simulink model "Islanding_case"  (R2024b)
settings: Solver=ode3  StartTime=0.0  StopTime=2.8  FixedStep=Ts  RelTol=1e-3  EnableMultiTasking=on
InitFcn:
  | Ts=100e-6;
  | Ts_Control=100e-6;
  | Ts_Power=100e-6;
  | tvv=0.1;
  | tr=1;
  | RelayEnableTime=1;
  | En_MC=1;
  | 
  | % ================= CHOOSE THE CASE HERE ==================
  | CaseNo    = 1;      % 1 = grid connected   2 = islanding   3 = fault during islanding
  | FaultType = 'none';   % 'none'  'LG'  'LL'  'LLG'  'LLL'  'LLLG'   (not used in case 2)
  | Qmismatch = 0;      % extra capacitive reactive power (% of 1.5 MW per load); try 1 in case 2 to see the inverter trip
  | % =========================================================
  | 
  | % ---- settings derived from the case (no need to edit)
  | switch CaseNo
  |     case 1, Tisland = 100; Pmismatch = 50; Tf = 2.0;   % grid + PV supply the load, fault at 2.0 s
  |     case 2, Tisland = 2.0; Pmismatch = 0;  Tf = 100;   % breakers open at 2.0 s, no fault
  |     case 3, Tisland = 2.0; Pmismatch = 0;  Tf = 2.3;   % breakers open at 2.0 s, fault at 2.3 s
  |     otherwise, error('CaseNo must be 1, 2 or 3');
  | end
  | FaultDur = 0.1;     % fault duration (s)
  | Tf_LG   = 100; Tf_LL = 100; Tf_LLG = 100; Tf_LLL = 100; Tf_LLLG = 100;   % 100 = never
  | switch upper(FaultType)
  |     case 'LG',   Tf_LG   = Tf;
  |     case 'LL',   Tf_LL   = Tf;
  |     case 'LLG',  Tf_LLG  = Tf;
  |     case 'LLL',  Tf_LLL  = Tf;
  |     case 'LLLG', Tf_LLLG = Tf;
  |     case 'NONE'
  |     otherwise, error('FaultType must be none, LG, LL, LLG, LLL or LLLG');
  | end
undefined symbols (not defined in the file or in its folder): DiscIntNeverNeededParam, Finit, Newton, Raphson, Tisland
libraries: simulink x33, spsOnDelayLib x17, powerlib_extras x11, eeGeneralControl x9, spsThreePhaseFaultLib x6, slpidlib x6, spsThreePhaseVIMeasurementLib x4, spsSampleandHoldLib x4, spsAlphaBetaZerotodq0Lib x4, spsThreePhaseSourceLib x4, spsThreePhaseBreakerLib x3, simulink_extras x3
(part 3 of 4)

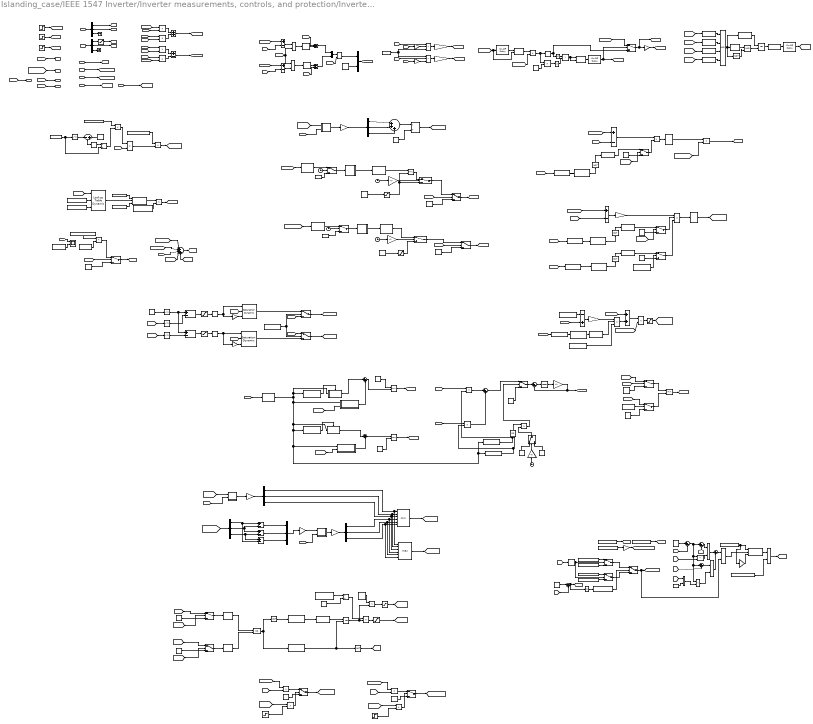
== system Islanding_case/IEEE 1547 Inverter/Inverter measurements, controls, and protection/Inverter control in positive sequence/Controls and grid support functions block ==
  note: |
      | |
      | |
      | |
      | |
      | |
      | |
      | |
      | |
      | |
      | |
      | |
      | |
      | |
      | |
      | |
      | |
      | |
      | |
      | |
      | |
      | |
      | |
      | |
      | |
      | |
      | |
      | |
      | |
      | |
      | |
      | |
      | |
      | |
      | |
      | |
      | |
      | |
      | |
      | |
      | |
      | |
      | |
      | |
      | |
      | |
      | |
      | |
      | |
      | |
      | |
      | |
      | |
      | |
      | |
      | |
  note: Group 2C Islanding Detection Function
  note: Enter Service Criteria
  note: Enter service
  note: Dynamic Voltage Support (DVS) in positive sequence
  note: Watt-Var Function
  note: Constant Q Function
  note: Constant PF Function
  note: |
      | |
      | |
      | |
      | |
      | |
      | |
      | |
      | |
      | |
      | |
      | |
      | |
      | |
      | |
      | |
      | |
      | |
      | |
      | |
  note: |
      | |
      | |
      | |
      | |
      | |
      | |
      | |
      | |
      | |
      | |
      | |
      | |
      | |
      | |
      | |
      | |
      | |
      | |
      | |
      | |
      | |
      | |
      | |
      | |
      | |
      | |
      | |
      | |
      | |
      | |
      | |
      | |
      | |
      | |
      | |
      | |
      | |
      | |
      | |
      | |
      | |
      | |
      | |
      | |
      | |
      | |
      | |
      | |
      | |
      | |
      | |
      | |
      | |
      | |
      | |
  note: Vca_rms
  note: Vbc_rms
  note: Vab_rms
  note: Vb_rms
  note: Vc_rms
  note: Vab
  note: Vca
  note: Vbc
  note: Va_rms
  note: If Volt-Var function is turned off, the inverter will function at unity power factor
  note: Momentary Cessation recover signal reset. Reset is 0 when momentary cessation ends and 1 during momentary cessation
  note: Volt-Var curve points
  note: Volt-watt curve points
  note: Output of the freq-watt control. Control to ensure that the output is either the active power adjustment due to under or over frequency
  note: Minimum of the active power generated from freq-watt control and volt-watt control
      | (PFV is the input to the power limiter)
  note: Active power adjustment for over frequency condition
  note: Active power adjustment for under frequency condition
  note: Maximum of phase to ground and phase to phase voltages as input to Momentary Cessation
  note: Minimum of phase to ground and phase to phase voltages as input to Momentary Cessation
  note: Momentary Cessation recovery ramp rate signal for active current
  note: Combine enter and exit Momentary Cessation signal into one control signal for active current
  note: Combine enter and exit Momentary Cessation signal into one control signal for reactive current
  note: Exit Momentary Cessation signal (Must be between 0 and 1)
  note: Enter Momentary Cessation signal
      | MC_sig is 0 when enter momentary cessation otherwise MC_sig is 1
  note: Multiply current references with MC_power_control to enter and exit Momentary Cessation
  note: Input to Momentary Cessation
  note: Momentary Cessation
  note: Freq-Watt Function
  note: Input to Volt-Watt and Volt-Var Function
  note: Volt-Watt Function
  note: Volt-Var Function
  note: Power limiter with Q priority
  note: Reactive power control
  note: Active power control
  note: Current controller
  note: Power calculation
  note: |
      | |
      | |
      | |
      | |
      | |
      | |
      | |
      | |
      | |
      | |
      | |
      | |
      | |
      | |
      | |
      | |
      | |
      | |
      | |
  note: |
      | |
      | |
      | |
      | |
      | |
      | |
      | |
      | |
      | |
      | |
      | |
      | |
      | |
      | |
      | |
      | |
      | |
      | |
      | |
      | |
      | |
      | |
      | |
      | |
      | |
      | |
      | |
      | |
      | |
      | |
      | |
      | |
      | |
      | |
      | |
      | |
      | |
      | |
      | |
      | |
      | |
      | |
      | |
      | |
      | |
      | |
      | |
      | |
      | |
      | |
      | |
      | |
      | |
      | |
      | |
  note: ==============================================================================================================================================================================================================================
  note: ========================================================================================================================================================================================================================================================
  note: ========================================================================================================================================================================================================================================================
  note: |
      | |
      | |
      | |
      | |
      | |
      | |
      | |
      | |
      | |
      | |
      | |
      | |
      | |
      | |
      | |
      | |
      | |
      | |
      | |
  note: |
      | |
      | |
      | |
      | |
      | |
      | |
      | |
      | |
      | |
      | |
      | |
      | |
      | |
      | |
      | |
      | |
      | |
      | |
      | |
  note: Inputs
  note: =============================================================================================================================================================================================================================================================================
  note: Pmin
  note: Pavailable
  note: |
      | |
      | |
      | |
      | |
      | |
      | |
      | |
      | |
      | |
      | |
      | |
      | |
      | |
      | |
      | |
      | |
      | |
      | |
      | |
  I_dq : Inport
  f : Inport  Port=2
  V_dq : Inport  Port=3
  Vpccpu : Inport  Port=4
  Vpcc : Inport  Port=5
  Idref_lim : Inport  Port=6
  Iqref_lim : Inport  Port=7
  -2 : Gain  Gain=Kpos  SaturateOnIntegerOverflow=on  OutDataTypeStr=Inherit: Same as input  ParamDataTypeStr=Inherit: Same as input
  -3 : Gain  Gain=-1  SaturateOnIntegerOverflow=on  OutDataTypeStr=Inherit: Same as input  ParamDataTypeStr=Inherit: Same as input
  -kd*L_ac : Gain  Gain=-kd*L_dec  SaturateOnIntegerOverflow=on  OutDataTypeStr=Inherit: Same as input  ParamDataTypeStr=Inherit: Same as input
  81U-2 Delay : spsOnDelayLib/On Delay  DelayType=On delay  delay=.016  ic=0  Ts=0
  81U-2 Delay1 : spsOnDelayLib/On Delay  DelayType=On delay  delay=.016  ic=0  Ts=0
  81U-2 Delay3 : spsOnDelayLib/On Delay  DelayType=Off delay  delay=0.016  ic=0  Ts=0
  81U-2 Delay4 : spsOnDelayLib/On Delay  DelayType=Off delay  delay=1/MC_recoveryrate  ic=0  Ts=0
  81U-2 Delay5 : spsOnDelayLib/On Delay  DelayType=Off delay  delay=0.016  ic=0  Ts=0
  81U-2 Delay6 : spsOnDelayLib/On Delay  DelayType=Off delay  delay=0.016  ic=0  Ts=0
  AND : Logic  Inputs=4  IconShape=distinctive  AllPortsSameDT=off  OutDataTypeStr=boolean
  AND1 : Logic  IconShape=distinctive  AllPortsSameDT=off  OutDataTypeStr=boolean
  Abs : Abs  SaturateOnIntegerOverflow=off
  Abs1 : Abs  SaturateOnIntegerOverflow=off
  Abs2 : Abs  SaturateOnIntegerOverflow=off
  Activate : Product  OutDataTypeStr=double  RndMeth=Zero
  Activate1 : Product  OutDataTypeStr=double  RndMeth=Zero
  Activate3 : Product  OutDataTypeStr=double  RndMeth=Zero
  CONST_Q_MOD_ENABLE : Constant  Value=CONST_Q_MODE_ENABLE
  Clock{,1..2,5..6} (5 alike) : Clock
  Compare To Constant : simulink/Logic and Bit Operations/Compare To Constant  relop=<  const=low_MC  OutDataTypeStr=boolean
  Compare To Constant1 : simulink/Logic and Bit Operations/Compare To Constant  relop=>  const=high_MC  OutDataTypeStr=boolean
  Compare To Constant2 : simulink/Logic and Bit Operations/Compare To Constant  relop=>  const=ES_V_LOW  OutDataTypeStr=boolean
  Compare To Constant3 : simulink/Logic and Bit Operations/Compare To Constant  relop=<  const=ES_V_HIGH  OutDataTypeStr=boolean
  Compare To Constant4 : simulink/Logic and Bit Operations/Compare To Constant  relop=>  const=ES_F_LOW  OutDataTypeStr=boolean
  Compare To Constant5 : simulink/Logic and Bit Operations/Compare To Constant  relop=<  const=ES_F_HIGH  OutDataTypeStr=boolean
  Compare To Constant6 : simulink/Logic and Bit Operations/Compare To Constant  relop=>  const=ES_DELAY  OutDataTypeStr=boolean
  Compare To Constant7 : simulink/Logic and Bit Operations/Compare To Constant  relop=<=  const=NomFreq  OutDataTypeStr=boolean
  Compare To Constant8 : simulink/Logic and Bit Operations/Compare To Constant  relop=<  const=GROUP2C_AI_F_TH  OutDataTypeStr=boolean
  Const : Constant
  Constant : Constant  Value=Pmin  SampleTime=-1
  Constant{1,3,6..7,9,13,15..16,32..34} (11 alike) : Constant  SampleTime=-1
  Constant10 : Constant  Value=MC_recoveryrate  SampleTime=-1
  Constant11 : Constant  Value=1/0.016  SampleTime=-1
  Constant12 : Constant  Value=0.999
  Constant14 : Constant  Value=0  SampleTime=-1
  Constant17 : Constant  Value=-1
  Constant18 : Constant  Value=GROUP2C_AI_LIMIT
  Constant19 : Constant  Value=GROUP2C_AI_DB
  Constant2 : Constant  Value=EnableVW  SampleTime=-1
  Constant20 : Constant  Value=GROUP2C_AI_DB
  Constant21 : Constant  Value=GROUP2C_AI_LIMIT
  Constant22 : Constant  Value=GROUP2C_AI_LG1
  Constant23 : Constant  Value=GROUP2C_AI_HG1
  Constant24 : Constant  Value=GROUP2C_AI_LG2
  Constant25 : Constant  Value=GROUP2C_AI_HG2
  Constant26 : Constant  Value=NomFreq
  Constant28 : Constant  Value=GROUP2C_AI_ENABLE
  Constant30 : Constant  Value=CONST_Q_ref
  Constant31 : Constant  Value=CONST_Q_ref
  Constant4 : Constant  Value=Pref  SampleTime=-1
  Constant5 : Constant  Value=3  SampleTime=-1
  Constant8 : Constant  Value=NomFreq
  ConstantPF : Constant  Value=Constant_PF
  Constant_PF_Excitation : Constant  Value=Constant_PF_Excitation
  Constant_PF_Mode_Enable : Constant  Value=Constant_PF_Mode_Enable
  Convert to PU1 : Gain  Gain=1/((RMSVnom*sqrt(3))*sqrt(2))  SaturateOnIntegerOverflow=on  OutDataTypeStr=Inherit: Same as input  ParamDataTypeStr=Inherit: Same as input
  Data Type Conversion{,1..5} (6 alike) : DataTypeConversion  OutDataTypeStr=double  SaturateOnIntegerOverflow=off  RndMeth=Floor
  Demux{,1..2,7,9,11} (6 alike) : Demux  Outputs=3
  Discrete PID Controller : slpidlib/PID Controller  Controller=PI  Form=Parallel  TimeDomain=Continuous-time  UseExternalTs=off  SampleTime=-1  IntegratorMethod=Forward Euler  FilterMethod=Forward Euler  ControllerParametersSource=internal  P=Kpi  I=Kii  UseKiTs=off  D=0  UseExternalDerivativeSource=off  N=100  UseFilter=on  TunerSelectOption=Transfer Function Based (PID Tuner App)  InitialConditionSource=internal  InitialConditionForIntegrator=0.65  InitialConditionForFilter=0  DifferentiatorICPrevScaledInput=0  ExternalReset=none  TrackingMode=off  Kt=1  LimitOutput=on  SatLimitsSource=internal  UpperSaturationLimit=1  LowerSaturationLimit=-1  LinearizeAsGain=off  AntiWindupMode=none  Kb=1  LimitIntegrator=off  UpperIntegratorSaturationLimit=inf  LowerIntegratorSaturationLimit=-inf  POutMin=[]  POutMax=[]  IOutMin=[]  IOutMax=[]  DOutMin=[]  DOutMax=[]  NOutMin=[]  NOutMax=[]  SumOutMin=[]  SumOutMax=[]  SaturationOutMin=[]  SaturationOutMax=[]  PParamMin=[]  PParamMax=[]  IParamMin=[]  IParamMax=[]  DParamMin=[]  DParamMax=[]  NParamMin=[]  NParamMax=[]  KbParamMin=[]  KbParamMax=[]  KtParamMin=[]  KtParamMax=[]  KbOutMin=[]  KbOutMax=[]  KtOutMin=[]  KtOutMax=[]  IntegratorOutMin=[]  IntegratorOutMax=[]  FilterOutMin=[]  FilterOutMax=[]  SumI1OutMin=[]  SumI1OutMax=[]  SumI2OutMin=[]  SumI2OutMax=[]  SumI3OutMin=[]  SumI3OutMax=[]  SumI4OutMin=[]  SumI4OutMax=[]  SumDOutMin=[]  SumDOutMax=[]  DifferentiatorOutMin=[]  DifferentiatorOutMax=[]  FilterDiffOutCoefMin=[]  FilterDiffOutCoefMax=[]  ReciprocalOutMin=[]  ReciprocalOutMax=[]  SumDenOutMin=[]  SumDenOutMax=[]  SumNumOutMin=[]  SumNumOutMax=[]  DivideOutMin=[]  DivideOutMax=[]  UdiffTsProdOutMin=[]  UdiffTsProdOutMax=[]  NTsProdOutMin=[]  NTsProdOutMax=[]  UintegralTsProdOutMin=[]  UintegralTsProdOutMax=[]  UngainTsProdOutMin=[]  UngainTsProdOutMax=[]  ClampingZeroOutDataTypeStr=Inherit: Inherit via back propagation  ClampingZeroOutMin=[]  ClampingZeroOutMax=[]  FilterDenConstantOutDataTypeStr=Inherit: Inherit via back propagation  FilterDenConstantOutMin=[]  FilterDenConstantOutMax=[]  PCopyOutDataTypeStr=Inherit: Inherit via back propagation  PCopyOutMin=[]  PCopyOutMax=[]  NCopyOutDataTypeStr=Inherit: Inherit via back propagation  NCopyOutMin=[]  NCopyOutMax=[]  IntegratorContinuousStateAttributes=''  IntegratorStateMustResolveToSignalObject=off  IntegratorRTWStateStorageClass=Auto  FilterContinuousStateAttributes=''  FilterStateMustResolveToSignalObject=off  FilterRTWStateStorageClass=Auto  ParallelPVariant=InternalParameters  IdealPVariant=Disabled  IVariant=InternalParameters  DVariant=Disabled  IntegratorVariant=Continuous  SatVariant=Enabled  AWVariant=Passthrough  PCopyVariant=Disabled  TRVariant=Disabled  FdbkBlocksVariant=Forward  IdealPFdbkVariant=Disabled  SatFdbkVariant=Disabled  DerivativeFilterVariant=Disabled  NVariant=Disabled  NCopyVariant=Disabled_SignalSpec  FilterICVariant=Disabled  IntegratorICVariant=InternalICs  ExternalResetVariant=Disabled  TRSumVariant=Passthrough  SumFdbkVariant=Disabled  SumVariant=Sum_PI  TsampFilterVariant=InternalTs  TsampNgainVariant=Passthrough  TsampIntegralVariant=Disabled_SignalSpec  ExternalSaturationOutDataTypeStr=Inherit: Same as second input  DerivativeSourceVariant=Disabled  PreIntVariant=InternalPreInt
  Discrete PID Controller1 : slpidlib/PID Controller  Controller=PI  Form=Parallel  TimeDomain=Continuous-time  UseExternalTs=off  SampleTime=-1  IntegratorMethod=Forward Euler  FilterMethod=Forward Euler  ControllerParametersSource=internal  P=Kpi  I=Kii  UseKiTs=off  D=0  UseExternalDerivativeSource=off  N=100  UseFilter=on  TunerSelectOption=Transfer Function Based (PID Tuner App)  InitialConditionSource=internal  InitialConditionForIntegrator=0  InitialConditionForFilter=0  DifferentiatorICPrevScaledInput=0  ExternalReset=none  TrackingMode=off  Kt=1  LimitOutput=on  SatLimitsSource=internal  UpperSaturationLimit=1  LowerSaturationLimit=-1  LinearizeAsGain=off  AntiWindupMode=none  Kb=1  LimitIntegrator=off  UpperIntegratorSaturationLimit=inf  LowerIntegratorSaturationLimit=-inf  POutMin=[]  POutMax=[]  IOutMin=[]  IOutMax=[]  DOutMin=[]  DOutMax=[]  NOutMin=[]  NOutMax=[]  SumOutMin=[]  SumOutMax=[]  SaturationOutMin=[]  SaturationOutMax=[]  PParamMin=[]  PParamMax=[]  IParamMin=[]  IParamMax=[]  DParamMin=[]  DParamMax=[]  NParamMin=[]  NParamMax=[]  KbParamMin=[]  KbParamMax=[]  KtParamMin=[]  KtParamMax=[]  KbOutMin=[]  KbOutMax=[]  KtOutMin=[]  KtOutMax=[]  IntegratorOutMin=[]  IntegratorOutMax=[]  FilterOutMin=[]  FilterOutMax=[]  SumI1OutMin=[]  SumI1OutMax=[]  SumI2OutMin=[]  SumI2OutMax=[]  SumI3OutMin=[]  SumI3OutMax=[]  SumI4OutMin=[]  SumI4OutMax=[]  SumDOutMin=[]  SumDOutMax=[]  DifferentiatorOutMin=[]  DifferentiatorOutMax=[]  FilterDiffOutCoefMin=[]  FilterDiffOutCoefMax=[]  ReciprocalOutMin=[]  ReciprocalOutMax=[]  SumDenOutMin=[]  SumDenOutMax=[]  SumNumOutMin=[]  SumNumOutMax=[]  DivideOutMin=[]  DivideOutMax=[]  UdiffTsProdOutMin=[]  UdiffTsProdOutMax=[]  NTsProdOutMin=[]  NTsProdOutMax=[]  UintegralTsProdOutMin=[]  UintegralTsProdOutMax=[]  UngainTsProdOutMin=[]  UngainTsProdOutMax=[]  ClampingZeroOutDataTypeStr=Inherit: Inherit via back propagation  ClampingZeroOutMin=[]  ClampingZeroOutMax=[]  FilterDenConstantOutDataTypeStr=Inherit: Inherit via back propagation  FilterDenConstantOutMin=[]  FilterDenConstantOutMax=[]  PCopyOutDataTypeStr=Inherit: Inherit via back propagation  PCopyOutMin=[]  PCopyOutMax=[]  NCopyOutDataTypeStr=Inherit: Inherit via back propagation  NCopyOutMin=[]  NCopyOutMax=[]  IntegratorContinuousStateAttributes=''  IntegratorStateMustResolveToSignalObject=off  IntegratorRTWStateStorageClass=Auto  FilterContinuousStateAttributes=''  FilterStateMustResolveToSignalObject=off  FilterRTWStateStorageClass=Auto  ParallelPVariant=InternalParameters  IdealPVariant=Disabled  IVariant=InternalParameters  DVariant=Disabled  IntegratorVariant=Continuous  SatVariant=Enabled  AWVariant=Passthrough  PCopyVariant=Disabled  TRVariant=Disabled  FdbkBlocksVariant=Forward  IdealPFdbkVariant=Disabled  SatFdbkVariant=Disabled  DerivativeFilterVariant=Disabled  NVariant=Disabled  NCopyVariant=Disabled_SignalSpec  FilterICVariant=Disabled  IntegratorICVariant=InternalICs  ExternalResetVariant=Disabled  TRSumVariant=Passthrough  SumFdbkVariant=Disabled  SumVariant=Sum_PI  TsampFilterVariant=InternalTs  TsampNgainVariant=Passthrough  TsampIntegralVariant=Disabled_SignalSpec  ExternalSaturationOutDataTypeStr=Inherit: Same as second input  DerivativeSourceVariant=Disabled  PreIntVariant=InternalPreInt
  Discrete PID Controller3 : slpidlib/PID Controller  Controller=PI  Form=Parallel  TimeDomain=Discrete-time  UseExternalTs=off  SampleTime=-1  IntegratorMethod=Backward Euler  FilterMethod=Forward Euler  ControllerParametersSource=internal  P=Kpp  I=Kip  UseKiTs=off  D=0  UseExternalDerivativeSource=off  N=100  UseFilter=on  TunerSelectOption=Transfer Function Based (PID Tuner App)  ZeroCross=off  InitialConditionSource=internal  InitialConditionForIntegrator=0  InitialConditionForFilter=0  DifferentiatorICPrevScaledInput=0  ExternalReset=none  TrackingMode=off  Kt=1  LimitOutput=on  SatLimitsSource=internal  UpperSaturationLimit=Imax  LowerSaturationLimit=-Imax  LinearizeAsGain=off  AntiWindupMode=back-calculation  Kb=1  LimitIntegrator=off  UpperIntegratorSaturationLimit=inf  LowerIntegratorSaturationLimit=-inf  POutMin=[]  POutMax=[]  IOutMin=[]  IOutMax=[]  DOutMin=[]  DOutMax=[]  NOutMin=[]  NOutMax=[]  SumOutMin=[]  SumOutMax=[]  SaturationOutMin=[]  SaturationOutMax=[]  PParamMin=[]  PParamMax=[]  IParamMin=[]  IParamMax=[]  DParamMin=[]  DParamMax=[]  NParamMin=[]  NParamMax=[]  KbParamMin=[]  KbParamMax=[]  KtParamMin=[]  KtParamMax=[]  KbOutMin=[]  KbOutMax=[]  KtOutMin=[]  KtOutMax=[]  IntegratorOutMin=[]  IntegratorOutMax=[]  FilterOutMin=[]  FilterOutMax=[]  SumI1OutMin=[]  SumI1OutMax=[]  SumI2OutMin=[]  SumI2OutMax=[]  SumI3OutMin=[]  SumI3OutMax=[]  SumI4OutMin=[]  SumI4OutMax=[]  SumDOutMin=[]  SumDOutMax=[]  DifferentiatorOutMin=[]  DifferentiatorOutMax=[]  FilterDiffOutCoefMin=[]  FilterDiffOutCoefMax=[]  ReciprocalOutMin=[]  ReciprocalOutMax=[]  SumDenOutMin=[]  SumDenOutMax=[]  SumNumOutMin=[]  SumNumOutMax=[]  DivideOutMin=[]  DivideOutMax=[]  UdiffTsProdOutMin=[]  UdiffTsProdOutMax=[]  NTsProdOutMin=[]  NTsProdOutMax=[]  UintegralTsProdOutMin=[]  UintegralTsProdOutMax=[]  UngainTsProdOutMin=[]  UngainTsProdOutMax=[]  ClampingZeroOutDataTypeStr=Inherit: Inherit via back propagation  ClampingZeroOutMin=[]  ClampingZeroOutMax=[]  FilterDenConstantOutDataTypeStr=Inherit: Inherit via back propagation  FilterDenConstantOutMin=[]  FilterDenConstantOutMax=[]  PCopyOutDataTypeStr=Inherit: Inherit via back propagation  PCopyOutMin=[]  PCopyOutMax=[]  NCopyOutDataTypeStr=Inherit: Inherit via back propagation  NCopyOutMin=[]  NCopyOutMax=[]  IntegratorContinuousStateAttributes=''  IntegratorStateMustResolveToSignalObject=off  IntegratorRTWStateStorageClass=Auto  FilterContinuousStateAttributes=''  FilterStateMustResolveToSignalObject=off  FilterRTWStateStorageClass=Auto  ParallelPVariant=InternalParameters  IdealPVariant=Disabled  IVariant=InternalParameters  DVariant=Disabled  IntegratorVariant=Discrete  SatVariant=Enabled  AWVariant=BackCalculation  PCopyVariant=Disabled  TRVariant=Disabled  FdbkBlocksVariant=Feedback  IdealPFdbkVariant=Passthrough  SatFdbkVariant=Enabled  DerivativeFilterVariant=Disabled  NVariant=Disabled  NCopyVariant=Disabled_SignalSpec  FilterICVariant=Disabled  IntegratorICVariant=InternalICs  ExternalResetVariant=Disabled  TRSumVariant=Passthrough  SumFdbkVariant=Enabled  SumVariant=Sum_PI  TsampFilterVariant=InternalTs  TsampNgainVariant=Passthrough  TsampIntegralVariant=Disabled_SignalSpec  ExternalSaturationOutDataTypeStr=Inherit: Same as second input  DerivativeSourceVariant=Disabled  PreIntVariant=InternalPreInt
  Discrete PID Controller6 : slpidlib/PID Controller  Controller=PI  Form=Parallel  TimeDomain=Discrete-time  UseExternalTs=off  SampleTime=-1  IntegratorMethod=Backward Euler  FilterMethod=Forward Euler  ControllerParametersSource=internal  P=Kpp  I=Kip  UseKiTs=off  D=0  UseExternalDerivativeSource=off  N=100  UseFilter=on  TunerSelectOption=Transfer Function Based (PID Tuner App)  ZeroCross=off  InitialConditionSource=internal  InitialConditionForIntegrator=0  InitialConditionForFilter=0  DifferentiatorICPrevScaledInput=0  ExternalReset=none  TrackingMode=off  Kt=1  LimitOutput=on  SatLimitsSource=internal  UpperSaturationLimit=Imax  LowerSaturationLimit=-Imax  LinearizeAsGain=off  AntiWindupMode=clamping  Kb=1  LimitIntegrator=off  UpperIntegratorSaturationLimit=inf  LowerIntegratorSaturationLimit=-inf  POutMin=[]  POutMax=[]  IOutMin=[]  IOutMax=[]  DOutMin=[]  DOutMax=[]  NOutMin=[]  NOutMax=[]  SumOutMin=[]  SumOutMax=[]  SaturationOutMin=[]  SaturationOutMax=[]  PParamMin=[]  PParamMax=[]  IParamMin=[]  IParamMax=[]  DParamMin=[]  DParamMax=[]  NParamMin=[]  NParamMax=[]  KbParamMin=[]  KbParamMax=[]  KtParamMin=[]  KtParamMax=[]  KbOutMin=[]  KbOutMax=[]  KtOutMin=[]  KtOutMax=[]  IntegratorOutMin=[]  IntegratorOutMax=[]  FilterOutMin=[]  FilterOutMax=[]  SumI1OutMin=[]  SumI1OutMax=[]  SumI2OutMin=[]  SumI2OutMax=[]  SumI3OutMin=[]  SumI3OutMax=[]  SumI4OutMin=[]  SumI4OutMax=[]  SumDOutMin=[]  SumDOutMax=[]  DifferentiatorOutMin=[]  DifferentiatorOutMax=[]  FilterDiffOutCoefMin=[]  FilterDiffOutCoefMax=[]  ReciprocalOutMin=[]  ReciprocalOutMax=[]  SumDenOutMin=[]  SumDenOutMax=[]  SumNumOutMin=[]  SumNumOutMax=[]  DivideOutMin=[]  DivideOutMax=[]  UdiffTsProdOutMin=[]  UdiffTsProdOutMax=[]  NTsProdOutMin=[]  NTsProdOutMax=[]  UintegralTsProdOutMin=[]  UintegralTsProdOutMax=[]  UngainTsProdOutMin=[]  UngainTsProdOutMax=[]  ClampingZeroOutDataTypeStr=Inherit: Inherit via back propagation  ClampingZeroOutMin=[]  ClampingZeroOutMax=[]  FilterDenConstantOutDataTypeStr=Inherit: Inherit via back propagation  FilterDenConstantOutMin=[]  FilterDenConstantOutMax=[]  PCopyOutDataTypeStr=Inherit: Inherit via back propagation  PCopyOutMin=[]  PCopyOutMax=[]  NCopyOutDataTypeStr=Inherit: Inherit via back propagation  NCopyOutMin=[]  NCopyOutMax=[]  IntegratorContinuousStateAttributes=''  IntegratorStateMustResolveToSignalObject=off  IntegratorRTWStateStorageClass=Auto  FilterContinuousStateAttributes=''  FilterStateMustResolveToSignalObject=off  FilterRTWStateStorageClass=Auto  ParallelPVariant=InternalParameters  IdealPVariant=Disabled  IVariant=InternalParameters  DVariant=Disabled  IntegratorVariant=Discrete  SatVariant=Enabled  AWVariant=DiscClampingParallel  PCopyVariant=Disabled  TRVariant=Disabled  FdbkBlocksVariant=Feedback  IdealPFdbkVariant=Passthrough  SatFdbkVariant=Passthrough  DerivativeFilterVariant=Disabled  NVariant=Disabled  NCopyVariant=Disabled_SignalSpec  FilterICVariant=Disabled  IntegratorICVariant=InternalICs  ExternalResetVariant=Disabled  TRSumVariant=Passthrough  SumFdbkVariant=Enabled  SumVariant=Sum_PI  TsampFilterVariant=InternalTs  TsampNgainVariant=Passthrough  TsampIntegralVariant=Disabled_SignalSpec  ExternalSaturationOutDataTypeStr=Inherit: Same as second input  DerivativeSourceVariant=Disabled  PreIntVariant=InternalPreInt
  Discrete-Time Integrator : DiscreteIntegrator  InitialCondition=Pref*OLRT_FW/2.3  SampleTime=Ts  ICPrevOutput=DiscIntNeverNeededParam  ICPrevScaledInput=DiscIntNeverNeededParam
  Divide : Product  Inputs=*/
  Divide1 : Product  Inputs=*/
  Divide2 : Product  Inputs=*/
  Edge Detector : spsEdgeDetectorLib/Edge Detector  model=Either  ic=0  Ts=-1
      settings: LibrarySourceBlock=sps_lib/Control/Edge Detector
  Enable Decoupling : Constant  Value=En_Dec
  GT1 : RelationalOperator  Operator=>  OutDataTypeStr=boolean  RndMeth=Simplest  InputSameDT=off
  GT2 : RelationalOperator  Operator=>  OutDataTypeStr=boolean  RndMeth=Simplest  InputSameDT=off
  GT3 : RelationalOperator  Operator=<  OutDataTypeStr=boolean  RndMeth=Simplest  InputSameDT=off
  Gain : Gain  Gain=1/NomFreq
  Gain1 : Gain  Gain=1/NomFreq
  Gain13 : Gain  Gain=sqrt(2)
  Gain15 : Gain  Gain=sqrt(2)
  Gain2 : Gain  Gain=-1
  Gain3 : Gain  Gain=-1
  Gain4 : Gain  Gain=2.3/OLRT_FW
  Gain5 : Gain  Gain=EnableVW
  Gain6 : Gain  Gain=sqrt(2)
  Gain7 : Gain  Gain=EnableVQ
  Gain8 : Gain  Gain=EnableFW
  Gain9 : Gain  Gain=-1
  If : If  IfExpression=u1 < 59.964  ShowElse=off
  If Action Subsystem : Subsystem  TreatAsAtomicUnit=on
  If Action Subsystem1 : Subsystem  TreatAsAtomicUnit=on
  If1 : If  IfExpression=u1> 50.036  ShowElse=off
  Integrator : Integrator  ExternalReset=rising  UpperSaturationLimit=1  LowerSaturationLimit=0
  Integrator1 : Integrator  ExternalReset=either  LimitOutput=on  UpperSaturationLimit=100  LowerSaturationLimit=-100
  Iqref limits : Saturate  UpperLimit=Imax  LowerLimit=-Imax
  Lookup Table Dynamic : simulink/Lookup Tables/Lookup Table Dynamic  LookUpMeth=Interpolation-Use End Values  OutDataType=fixdt('double')  OutScaling=[]  OutputDataTypeScalingMode=Specify via dialog  OutDataTypeStr=fixdt('double')  DoSatur=off
  Low-Pass Filter (Discrete or Continuous) : eeGeneralControl/Low-Pass Filter (Discrete or Continuous)  K=1  T=0.1  B=inf  A=-inf  init_option=Inherited from block input  x0=0  Ts=-1
  Low-Pass Filter (Discrete or Continuous)4 : eeGeneralControl/Low-Pass Filter (Discrete or Continuous)  K=1  T=0.1  B=inf  A=-inf  init_option=Inherited from block input  x0=0  Ts=-1
  Low-Pass Filter (Discrete or Continuous)6 : eeGeneralControl/Low-Pass Filter (Discrete or Continuous)  K=1  T=OLRT_VWatt/2.3  B=inf  A=-inf  init_option=Inherited from block input  x0=0  Ts=-1
  Low-Pass Filter (Discrete or Continuous)7 : eeGeneralControl/Low-Pass Filter (Discrete or Continuous)  K=1  T=0.1  B=inf  A=-inf  init_option=Inherited from block input  x0=0  Ts=-1
  Low-Pass Filter (Discrete or Continuous)8 : eeGeneralControl/Low-Pass Filter (Discrete or Continuous)  K=1  T=OLRT_Vvar/2.3  B=inf  A=-inf  init_option=Inherited from block input  x0=0  Ts=-1
  MC_Enable : Step  Time=En_MC  SampleTime=0
  MC_Enable1 : Step  Time=En_MC  SampleTime=0
  Math Function2 : Math  Operator=square  SignedPower=on
  Math Function4 : Math  Operator=square  SignedPower=on
  Math Function5 : Math  Operator=square  SignedPower=on
  Min : MinMax  Inputs=2
  Min1 : MinMax  Inputs=2
  Min4 : MinMax  Inputs=6
  Min5 : MinMax  Function=max  Inputs=6
  MinMax2 : MinMax  Inputs=2
  MinMax3 : MinMax  Function=max  Inputs=2
  Multiply : Product
  Mux : Mux  Inputs=3
  Mux1 : Mux  Inputs=2
  Mux2 : Mux  Inputs=2
  NOT{,1..5} (6 alike) : Logic  Operator=NOT  IconShape=distinctive  AllPortsSameDT=off  OutDataTypeStr=boolean
  OF : simulink/Logic and Bit Operations/Compare To Constant  relop=>=  const=NomFreq+dbOF  OutDataTypeStr=boolean  ZeroCross=off
  OR : Logic  Operator=OR  IconShape=distinctive  AllPortsSameDT=off  OutDataTypeStr=boolean
  OR1 : Logic  Operator=OR  IconShape=distinctive  AllPortsSameDT=off  OutDataTypeStr=boolean
  On-Off Delay : eeGeneralControl/On-Off Delay  LabelModeActiveChoice=Discrete  Td_on=0  Td_off=10000  IC=0  Ts=Ts
  On-Off Delay1 : eeGeneralControl/On-Off Delay  LabelModeActiveChoice=Discrete  Td_on=0.1  Td_off=0.1  IC=0  Ts=Ts
  On-Off Delay2 : eeGeneralControl/On-Off Delay  LabelModeActiveChoice=Discrete  Td_on=0  Td_off=10000  IC=0  Ts=Ts
  One1 : Constant
  One7 : Constant
  Ppre over freq : Subsystem
  Ppre under freq : Subsystem
  Pref limits : Saturate  UpperLimit=1  LowerLimit=-1
  Product{,1..12,14..22,24} (23 alike) : Product
  Product13 : Product  Inputs=3
  Product23 : Product  Inputs=3
  "Q priority " : Constant
  QP_CURVE_Q3_ASP : Constant  Value=QP_CURVE_Q3_ASP
  QP_CURVE_Q3_GEN : Constant  Value=QP_CURVE_Q3_GEN
  QP_MODE_ENABLE : Constant  Value=QP_MODE_ENABLE
  Qref limits : Saturate  UpperLimit=0.44  LowerLimit=-0.44
  RMS1 : Subsystem  AncestorBlock=|  DialogController=POWERSYS.PowerSysDialog  mask(Discrete RMS value){Mag_Init=0, Ts=Ts}
      | powerlib_extras/Discrete
      | Measurements/Discrete 
      | RMS value
      mask prompts: Mag_Init "Initial magnitude of input:"; Ts "Sample time:"
      mask help:
      | Measure the true root mean square (RMS) value of a signal.
      |
      | To measure the RMS value of the fundamental component, use instead the Discrete Fourier block and divide its output by sqrt(2).
      mask init:
      | power_initmask();
      mask Help: web(psbhelp)
      mask Display: disp('RMS\n(discrete)')
  RMS6 : Subsystem  AncestorBlock=|  DialogController=POWERSYS.PowerSysDialog  mask(Discrete RMS value){Mag_Init=0, Ts=Ts}
      | powerlib_extras/Discrete
      | Measurements/Discrete 
      | RMS value
      mask prompts: Mag_Init "Initial magnitude of input:"; Ts "Sample time:"
      mask help:
      | Measure the true root mean square (RMS) value of a signal.
      |
      | To measure the RMS value of the fundamental component, use instead the Discrete Fourier block and divide its output by sqrt(2).
      mask init:
      | power_initmask();
      mask Help: web(psbhelp)
      mask Display: disp('RMS\n(discrete)')
  RMS9 : Subsystem  AncestorBlock=|  DialogController=POWERSYS.PowerSysDialog  mask(Discrete RMS value){Mag_Init=0, Ts=Ts}
      | powerlib_extras/Discrete
      | Measurements/Discrete 
      | RMS value
      mask prompts: Mag_Init "Initial magnitude of input:"; Ts "Sample time:"
      mask help:
      | Measure the true root mean square (RMS) value of a signal.
      |
      | To measure the RMS value of the fundamental component, use instead the Discrete Fourier block and divide its output by sqrt(2).
      mask init:
      | power_initmask();
      mask Help: web(psbhelp)
      mask Display: disp('RMS\n(discrete)')
  Rate Limiter : RateLimiter  RisingSlewLimit=ES_RAMP_RATE  FallingSlewLimit=-ES_RAMP_RATE  SampleTimeMode=inherited
  Sample and Hold1 : spsSampleandHoldLib/Sample and Hold  ic=0  Ts=Ts
      settings: LibrarySourceBlock=|
      | sps_lib/Control/Sample and
      | Hold
  Sample and Hold2 : spsSampleandHoldLib/Sample and Hold  ic=0  Ts=0
      settings: LibrarySourceBlock=|
      | sps_lib/Control/Sample and
      | Hold
  Saturation : Saturate  UpperLimit=1  LowerLimit=0
  Saturation Dynamic{2..3,6..7} (4 alike) : simulink/Discontinuities/Saturation Dynamic  OutMin=[]  OutMax=[]  OutDataTypeStr=Inherit: Same as second input  OutDataType=fixdt(1, 16)  OutScaling=2^-10  DoSatur=off
  Saturation3 : Saturate  UpperLimit=inf  LowerLimit=0
  Saturation4 : Saturate  UpperLimit=inf  LowerLimit=0
  Saturation5 : Saturate  UpperLimit=1  LowerLimit=0
  Scope10 : Scope  NumInputPorts=2
  Smax : Constant
  Sqrt2 : Sqrt
  Sqrt3 : Sqrt
  Sqrt4 : Sqrt
  Square : Math  Operator=square  SignedPower=on
  Step @ t=0.05s2 : Step  Time=0.05  SampleTime=0
  "Step @ t=0.5s " : Step  Time=0.5  SampleTime=0
  Step @ t=0.5s 2 : Step  Time=En_MC  After=EnableMC  SampleTime=0
  Subtract : Sum  Inputs=+-
  Subtract1 : Sum  Inputs=+-
  Subtract2 : Sum  Inputs=+-
  Subtract3 : Sum  Inputs=-+
  Sum{,11,14,21..22} (5 alike) : Sum  Inputs=|++
  Sum{1,3..4,7..8,18..19} (7 alike) : Sum  Inputs=+-
  Sum10 : Sum  Inputs=|+++++
  Sum13 : Sum  Inputs=|+-
  Sum15 : Sum  Inputs=|+++
  Sum{5..6,16,27} (4 alike) : Sum
  Sum20 : Sum  Inputs=|+-
  Sum23 : Sum  Inputs=|-+
  Sum26 : Sum  Inputs=-+
  Sum9 : Sum  Inputs=|+-
  Switch{,6,10..11,14..15,21..23} (9 alike) : Switch  Criteria=u2 > Threshold  Threshold=0.5  SaturateOnIntegerOverflow=off  InputSameDT=off
  Switch{1,4..5,7,9,17} (6 alike) : Switch  Threshold=0.5  SaturateOnIntegerOverflow=off  InputSameDT=off
  Switch12 : Switch  Criteria=u2 > Threshold  Threshold=En_VWatt  SaturateOnIntegerOverflow=off  InputSameDT=off
  Switch13 : Switch  Threshold=tvv  SaturateOnIntegerOverflow=off  InputSameDT=off
  Switch16 : Switch  Threshold=0.5  RndMeth=Zero  SaturateOnIntegerOverflow=off  InputSameDT=off
  Switch18 : Switch  Threshold=1  SaturateOnIntegerOverflow=off  InputSameDT=off
  Switch19 : Switch  Threshold=1  SaturateOnIntegerOverflow=off  InputSameDT=off
  Switch2 : Switch  Criteria=u2 > Threshold  Threshold=En_VVar  SaturateOnIntegerOverflow=off  InputSameDT=off
  Switch20 : Switch  Threshold=1  SaturateOnIntegerOverflow=off  InputSameDT=off
  Switch3 : Switch  Threshold=tvv  SaturateOnIntegerOverflow=off  InputSameDT=off
  Switch8 : Switch  Criteria=u2 > Threshold  Threshold=En_FW  SaturateOnIntegerOverflow=off  InputSameDT=off
  Terminator2 : Terminator
  Terminator3 : Terminator
  UF : simulink/Logic and Bit Operations/Compare To Constant  relop=<=  const=NomFreq-dbUF  OutDataTypeStr=boolean  ZeroCross=off
  UV1 : simulink/Logic and Bit Operations/Compare To Constant  relop=<  const=0.5  OutDataTypeStr=boolean  ZeroCross=off
  UV2 : simulink/Logic and Bit Operations/Compare To Constant  relop=<  const=DVS_Threshold  OutDataTypeStr=boolean  ZeroCross=off
  UV3 : simulink/Logic and Bit Operations/Compare To Constant  relop=<  const=0.5  OutDataTypeStr=boolean  ZeroCross=off
  UV4 : simulink/Logic and Bit Operations/Compare To Constant  relop=<  const=DVS_Threshold  OutDataTypeStr=boolean  ZeroCross=off
  U_0 : Constant  Value=0
  VAR setpoints : Constant  Value=[QP_CURVE_Q3_ASP QP_CURVE_Q2_ASP QP_CURVE_Q1_ASP QP_CURVE_Q1_GEN QP_CURVE_Q2_GEN QP_CURVE_Q3_GEN]
  VV controller : Subsystem
  VW controller : Subsystem
  Vd*Id : Product
  Vd*Iq : Product
  Vdlimit : Saturate  UpperLimit=2  LowerLimit=0
  Vq*Id : Product
  Vq*Iq : Product
  Watt setpoints : Constant  Value=[QP_CURVE_P3_ASP QP_CURVE_P2_ASP QP_CURVE_P1_ASP QP_CURVE_P1_GEN QP_CURVE_P2_GEN QP_CURVE_P3_GEN]
  Zero{,1..2,7..8} (5 alike) : Constant  Value=0
  Zero3 : Constant  Value=DVS_ENABLE
  Zero4 : Constant  Value=Vref_DVS
  Zero5 : Constant  Value=Pref
  Zero6 : Constant  Value=DVS_ENABLE
  f*Id : Product  Inputs=3  OutDataTypeStr=double  RndMeth=Zero
  f*Iq : Product  Inputs=3  OutDataTypeStr=double  RndMeth=Zero
  gain1 : Gain  Gain=-1
  gain2 : Gain  Gain=-1
  kd*L_ac : Gain  Gain=kd*L_dec  SaturateOnIntegerOverflow=on  OutDataTypeStr=Inherit: Same as input  ParamDataTypeStr=Inherit: Same as input
  U_dq : Outport  VectorParamsAs1DForOutWhenUnconnected=off
  MC : Outport  Port=2  VectorParamsAs1DForOutWhenUnconnected=off
  Iqposref : Outport  Port=3  VectorParamsAs1DForOutWhenUnconnected=off
  Idposref : Outport  Port=4  VectorParamsAs1DForOutWhenUnconnected=off
  Vmin : Outport  Port=5  VectorParamsAs1DForOutWhenUnconnected=off
  wires:
  Switch17/1 -> Min1/1  "Pref"
  [P_UF_OF] -> Switch17/1
  Zero8/1 -> Switch17/3
  [PQ_En] -> Switch17/2
  Switch6/1 -> Min1/2
  Constant16/1 -> Switch6/3
  [Pcom] -> Switch6/1
  Constant2/1 -> Switch6/2
  [PQ_En] -> Switch5/2
  Switch5/1 -> [Qref_CQ]  "Qref"
  Zero7/1 -> Switch5/3
  Abs2/1 -> GT1/1
  Abs1/1 -> GT1/2
  Product1/1 -> Abs1/1
  Switch23/1 -> Product13/3
  -2/1 -> Product23/1
  Switch22/1 -> Product13/2
  Vdlimit/1 -> [V_d]
  [Vmin] -> Vmin/1
  Product18/1 -> Sum21/1
  Constant18/1 -> gain2/1, Saturation Dynamic7/1
  [db2] -> Sum20/2
  Constant23/1 -> Switch18/3
  [db1] -> Sum22/2
  Constant26/1 -> Sum23/1
  [f] -> Compare To Constant7/1
  Constant22/1 -> Switch18/1
  Constant8/1 -> Sum13/1
  Constant24/1 -> Switch19/1
  Constant20/1 -> [db2]
  Abs/1 -> Compare To Constant8/1
  Constant28/1 -> Product21/2
  Saturation Dynamic7/1 -> Product21/1
  Product19/1 -> Sum21/2
  gain2/1 -> Saturation Dynamic7/3
  Sum13/1 -> Sum20/1, GT2/1, Sum22/1, GT3/1
  Product21/1 -> [Q_AI]
  Product22/1 -> Saturation Dynamic7/2
  Compare To Constant8/1 -> Switch20/2
  Switch18/1 -> Switch20/1
  gain1/1 -> [GROUP2C_AI_N_LIMIT]
  [f] -> Sum23/2
  Constant21/1 -> gain1/1
  Sum21/1 -> Product22/1
  Sum23/1 -> [dif_f], Abs/1
  Compare To Constant7/1 -> Switch18/2, Switch19/2
  Switch20/1 -> [GROUP2C_gain], Product22/2
  Constant19/1 -> [db1]
  Constant25/1 -> Switch19/3
  [db1] -> Product20/1
  Switch19/1 -> Switch20/3
  [db2] -> GT2/2
  Constant17/1 -> Product20/2
  Sum22/1 -> Product19/1
  Product20/1 -> GT3/2
  GT3/1 -> Product19/2
  Sum20/1 -> Product18/1
  GT2/1 -> Product18/2
  [f] -> Sum13/2
  Integrator1/1 -> Compare To Constant6/1
  [f] -> Compare To Constant5/1
  Compare To Constant3/1 -> AND/2
  Compare To Constant5/1 -> AND/4
  Compare To Constant4/1 -> AND/3
  [Vmin] -> Compare To Constant2/1
  [Vmax] -> Compare To Constant3/1
  AND/1 -> Edge Detector/1, NOT1/1, Data Type Conversion3/1
  Compare To Constant6/1 -> On-Off Delay/1
  AND1/1 -> Integrator1/2
  Edge Detector/1 -> AND1/1
  [f] -> Compare To Constant4/1
  Compare To Constant2/1 -> AND/1
  NOT1/1 -> AND1/2
  On-Off Delay/1 -> [ES_ACTIVE]
  Data Type Conversion3/1 -> Integrator1/1
  Zero4/1 -> Sum26/1
  Zero3/1 -> Product23/3
  [V_d] -> Sum26/2
  Iqref_lim/1 -> [I_q_refLim]
  Idref_lim/1 -> [I_d_refLim]
  [I_d_ref] -> Idposref/1
  [I_q_ref] -> Iqposref/1
  [MC_power_controlQ] -> MC/1
  Iqref limits/1 -> [I_q_ref]
  81U-2 Delay6/1 -> Data Type Conversion5/1
  81U-2 Delay5/1 -> NOT3/1
  81U-2 Delay3/1 -> NOT2/1
  [MC_power_controlQ] -> Product24/2
  Sum27/1 -> Product24/1
  Product24/1 -> Iqref limits/1
  Data Type Conversion5/1 -> Product23/2
  UV4/1 -> 81U-2 Delay6/1
  [Vmin] -> UV4/1
  Product23/1 -> Sum27/2
  Sum26/1 -> -2/1
  [I_q_ref_QC] -> Sum27/1
  [Vmin] -> UV2/1
  NOT3/1 -> Data Type Conversion4/1
  UV2/1 -> 81U-2 Delay5/1
  Zero6/1 -> Switch23/2
  Constant34/1 -> Switch23/3
  Data Type Conversion4/1 -> Switch23/1
  Data Type Conversion2/1 -> Switch22/1
  [MC_enable] -> Switch22/2
  Constant33/1 -> Switch22/3
  Data Type Conversion1/1 -> Switch21/1
  Switch21/1 -> Product12/2
  Constant32/1 -> Switch21/3
  [MC_enable] -> Switch21/2
  [Qcom] -> Sum10/5
  [ES_ACTIVE] -> Sample and Hold1/2, On-Off Delay1/1
  Product3/1 -> Product6/2
  Constant30/1 -> Scope10/2
  [Qref] -> Scope10/1
  Product16/1 -> [Q_ref_PQ]
  QP_MODE_ENABLE/1 -> Product16/2
  Saturation Dynamic6/1 -> Product16/1
  QP_CURVE_Q3_GEN/1 -> Saturation Dynamic6/3
  QP_CURVE_Q3_ASP/1 -> Saturation Dynamic6/1
  Lookup Table Dynamic/1 -> Saturation Dynamic6/2
  Watt setpoints/1 -> Lookup Table Dynamic/2
  VAR setpoints/1 -> Lookup Table Dynamic/3
  [PpccPu] -> Lookup Table Dynamic/1
  Product8/1 -> Switch5/1
  CONST_Q_MOD_ENABLE/1 -> Product8/1
  Constant31/1 -> Product8/2
  Sum10/1 -> [Qref]
  [Qref_CQ] -> Sum10/4
  [Q_AI] -> Sum10/3
  [Qref_PF] -> Sum10/2
  [Q_ref_PQ] -> Sum10/1
  [PpccPu] -> Product3/2
  Constant_PF_Mode_Enable/1 -> Product6/1
  Product6/1 -> [Qref_PF]
  Product2/1 -> Product3/1
  Constant_PF_Excitation/1 -> Product2/1
  Divide2/1 -> Product2/2
  ConstantPF/1 -> Square/1, Divide2/2
  Sqrt4/1 -> Divide2/1
  Subtract3/1 -> Sqrt4/1
  Const/1 -> Subtract3/2
  Square/1 -> Subtract3/1
  Gain9/1 -> [n_P_max]
  Switch16/1 -> Gain9/1, [P_max]
  [Pcom_limited] -> Switch16/1
  On-Off Delay2/1 -> [ES_status], Switch16/2
  Sample and Hold2/1 -> On-Off Delay2/1
  GT1/1 -> Sample and Hold2/1, Sample and Hold2/2
  Rate Limiter/1 -> Switch16/3, Abs2/1
  Constant12/1 -> Product1/2
  Product/1 -> Rate Limiter/1, Product1/1
  [Pcom_limited] -> Product/2
  Sample and Hold1/1 -> Product/1
  On-Off Delay1/1 -> Sample and Hold1/1
  81U-2 Delay4/1 -> NOT/1
  Switch8/1 -> Product7/2
  Constant15/1 -> Switch8/1
  Constant14/1 -> Switch8/3
  Gain8/1 -> Switch8/2
  Clock2/1 -> Gain8/1
  Gain7/1 -> Switch2/2
  Gain5/1 -> Switch12/2
  Sum9/1 -> Discrete-Time Integrator/1
  Switch/1 -> Sum9/1
  Gain4/1 -> [P_UF_OF], Sum9/2
  Mux/1 -> Convert to PU1/1
  Gain13/1 -> Demux7/1
  Demux11/1 -> Min4/4, Min5/4
  Demux9/3 -> Subtract2/1, Subtract1/2
  [f] -> RMS9/2(Freq)
  Demux7/2 -> Min4/2, Min5/2
  [VPCC_inv_pu] -> RMS6/1(In)
  Subtract1/1 -> Mux/2
  [f] -> RMS6/2(Freq)
  Min4/1 -> [Vmin]
  Demux7/3 -> Min4/3, Min5/3
  Demux7/1 -> Min4/1, Min5/1
  Subtract2/1 -> Mux/3
  Convert to PU1/1 -> RMS9/1(In)
  Demux11/2 -> Min4/5, Min5/5
  Demux9/2 -> Subtract1/1, Subtract/2
  Demux11/3 -> Min4/6, Min5/6
  Gain15/1 -> Demux11/1
  [VPCC_inv] -> Demux9/1
  Min5/1 -> [Vmax]
  RMS6/1(RMS) -> Gain13/1
  Demux9/1 -> Subtract/1, Subtract2/2
  RMS9/1(RMS) -> Gain15/1
  Subtract/1 -> Mux/1
  Step @ t=0.5s 2/1 -> [MC_enable]
  Demux1/1 -> Sum15/1
  [VPCC_inv_pu] -> RMS1/1(In)
  Divide/1 -> [Vrms_avg]
  Gain6/1 -> Demux1/1
  [f] -> RMS1/2(Freq)
  Constant5/1 -> Divide/2
  Demux1/2 -> Sum15/2
  Sum15/1 -> Divide/1
  Demux1/3 -> Sum15/3
  RMS1/1(RMS) -> Gain6/1
  Constant1/1 -> Divide1/2
  Constant10/1 -> Divide1/1
  Saturation5/1 -> [MC_recover]
  Divide1/1 -> Product11/1
  Product11/1 -> Saturation5/1
  Saturation/1 -> [MC_recoverQ]
  [MC_sig] -> Product17/2
  [MC_recoverQ] -> Product17/1
  [MC_enable] -> Product15/1
  MC_Enable1/1 -> Product15/2
  Product15/1 -> Switch15/2
  Product17/1 -> Switch15/1
  Switch15/1 -> [MC_power_controlQ]
  Constant13/1 -> Switch15/3
  Product14/1 -> Saturation/1
  Constant11/1 -> Product14/1
  NOT2/1 -> Data Type Conversion2/1
  NOT/1 -> Data Type Conversion1/1
  Sum19/1 -> Product12/1
  Vpcc/1 -> [VPCC_inv]
  NOT4/1 -> 81U-2 Delay1/1
  Data Type Conversion/1 -> Integrator/1
  81U-2 Delay1/1 -> Data Type Conversion/1
  Integrator/1 -> Product11/2, Product14/2
  MC_Enable/1 -> Product10/2
  Switch14/1 -> [MC_power_control]
  [MC_enable] -> Product10/1
  Product10/1 -> Switch14/2
  Constant9/1 -> Switch14/3
  Product9/1 -> Switch14/1
  [MC_recover] -> Product9/1
  [MC_sig] -> Product9/2
  Compare To Constant1/1 -> OR1/1
  Compare To Constant/1 -> OR1/2
  NOT5/1 -> [MC_sig]
  81U-2 Delay/1 -> Integrator/2, NOT5/1
  OR1/1 -> NOT4/1, 81U-2 Delay/1
  Switch11/1 -> Compare To Constant/1
  Switch10/1 -> Compare To Constant1/1
  [Vmin] -> Switch11/1
  Constant7/1 -> Switch11/3
  [MC_enable] -> Switch11/2
  [Vmax] -> Switch10/1
  Constant6/1 -> Switch10/3
  [MC_enable] -> Switch10/2
  Discrete PID Controller3/1 -> [I_q_ref_QC]
  UV3/1 -> 81U-2 Delay3/1
  [Vmin] -> UV3/1
  Product13/1 -> Discrete PID Controller3/1
  -3/1 -> Product13/1
  Multiply/1 -> [I_d_ref]
  [MC_power_control] -> Multiply/2
  Discrete PID Controller6/1 -> Multiply/1  "I_d_ref"
  UV1/1 -> 81U-2 Delay4/1
  [Vmin] -> UV1/1
  Product12/1 -> Discrete PID Controller6/1
  [QpccPu] -> Sum18/2
  Sum18/1 -> -3/1
  [PpccPu] -> Sum19/2
  [Qcom_limited] -> Sum18/1
  [P_max] -> Sum19/1
  Vpccpu/1 -> [VPCC_inv_pu]
  Discrete-Time Integrator/1 -> Gain4/1
  Product7/1 -> Switch/2
  OR/1 -> Product7/1
  [PpccPu] -> Ppre under freq/2(Ppu)
  [f] -> Low-Pass Filter (Discrete or Continuous)/1
  If1/1 -> If Action Subsystem1/Action
  If/1 -> If Action Subsystem/Action
  Low-Pass Filter (Discrete or Continuous)/1 -> Ppre under freq/1(f), UF/1, OF/1, Ppre over freq/1(f), If1/1, If Action Subsystem1/1(f), If Action Subsystem/1(f), If/1
  Min1/1 -> [PFV]
  Sum14/1 -> Switch/1
  Constant4/1 -> Switch/3
  OF/1 -> Product5/2, OR/2
  UF/1 -> Product4/2, OR/1
  Product5/1 -> Sum14/2
  Product4/1 -> Sum14/1
  [P_UF] -> Product4/1
  [P_OF] -> Product5/1
  [PpccPu] -> Ppre over freq/2(Ppu)
  Ppre over freq/1(Ppre) -> Sum11/2
  Ppre under freq/1(Ppre) -> Sum/2
  Constant3/1 -> MinMax2/1
  If Action Subsystem1/1(Pdelta) -> Sum11/1
  If Action Subsystem/1(Pdelta) -> Sum/1
  Sum11/1 -> MinMax3/1
  Sum/1 -> MinMax2/2
  MinMax3/1 -> [P_OF]
  Constant/1 -> MinMax3/2
  MinMax2/1 -> [P_UF]
  Low-Pass Filter (Discrete or Continuous)7/1 -> Switch3/1
  Switch2/1 -> Switch7/1
  Switch12/1 -> Switch1/1
  Min/1 -> Switch12/1
  Pref limits/1 -> Min/2, Switch12/3
  Clock5/1 -> Gain5/1
  [Vrms_avg] -> Low-Pass Filter (Discrete or Continuous)4/1
  One7/1 -> Switch13/3
  VW controller/1(Pref) -> Low-Pass Filter (Discrete or Continuous)6/1
  Clock6/1 -> Switch13/2
  Low-Pass Filter (Discrete or Continuous)6/1 -> Min/1
  Switch13/1 -> VW controller/1(V)
  Low-Pass Filter (Discrete or Continuous)4/1 -> Switch13/1
  Zero5/1 -> Pref limits/1
  Zero1/1 -> Qref limits/1
  Gain1/1 -> f*Id/3
  Gain/1 -> f*Iq/2
  [Vrms_avg] -> Low-Pass Filter (Discrete or Continuous)7/1
  Switch3/1 -> VV controller/1(V)
  Clock1/1 -> Switch3/2
  One1/1 -> Switch3/3
  Low-Pass Filter (Discrete or Continuous)8/1 -> Switch2/1
  VV controller/1(Qref) -> Low-Pass Filter (Discrete or Continuous)8/1
  Clock/1 -> Gain7/1
  [I_q_refLim] -> Sum4/1
  Switch4/1 -> [Pcom_limited]
  Switch1/1 -> [Pcom]  "Pref"
  [PQ_En] -> Switch1/2
  Zero2/1 -> Switch1/3
  Demux2/1 -> Vdlimit/1
  [QpccPu] -> Math Function4/1
  Switch9/1 -> [Qcom_limited]
  Sum16/1 -> [PpccPu]
  Sum1/1 -> [QpccPu]
  Switch7/1 -> [Qcom]  "Qref"
  Sum6/1 -> Mux2/2
  Demux2/3 -> Terminator3/1
  Demux/3 -> Terminator2/1
  [I_q] -> f*Iq/1
  [I_d] -> f*Id/2
  [PI_En] -> Activate/2, Activate1/1
  Step @ t=0.05s2/1 -> [PI_En]
  Discrete PID Controller/1 -> Sum5/2
  [PI_En] -> Activate3/2
  V_dq/1 -> Demux2/1
  Demux2/2 -> [V_q]
  Mux2/1 -> Activate3/1
  [ddec] -> Sum5/1
  [qdec] -> Sum6/2
  kd*L_ac/1 -> [qdec]
  -kd*L_ac/1 -> [ddec]
  Enable Decoupling/1 -> f*Id/1, f*Iq/3
  f*Id/1 -> kd*L_ac/1
  [f] -> Gain/1
  f*Iq/1 -> -kd*L_ac/1
  Discrete PID Controller1/1 -> Sum6/1
  [f] -> Gain1/1
  f/1 -> [f]
  Sum5/1 -> Mux2/1
  Sum4/1 -> Activate1/2
  Activate1/1 -> Discrete PID Controller1/1
  Activate/1 -> Discrete PID Controller/1
  Sum3/1 -> Activate/1
  Demux/2 -> [I_q]
  Demux/1 -> [I_d]
  I_dq/1 -> Demux/1
  [U_dq] -> U_dq/1
  [I_q] -> Sum4/2
  [I_d] -> Sum3/2
  Activate3/1 -> Mux1/1
  U_0/1 -> Mux1/2
  Mux1/1 -> [U_dq]
  [I_d_refLim] -> Sum3/1
  [V_q] -> Vq*Iq/1
  [I_q] -> Vq*Iq/2
  [I_d] -> Vd*Id/2
  [V_d] -> Vd*Id/1
  Vd*Id/1 -> Sum16/1
  Vq*Iq/1 -> Sum16/2
  Vd*Iq/1 -> Sum1/2
  Vq*Id/1 -> Sum1/1
  [I_d] -> Vq*Id/2
  [V_q] -> Vq*Id/1
  [I_q] -> Vd*Iq/1
  [V_d] -> Vd*Iq/2
  "Step @ t=0.5s "/1 -> [PQ_En]
  [PQ_En] -> Switch7/2
  Zero/1 -> Switch7/3
  Smax/1 -> Math Function2/1
  Math Function4/1 -> Sum8/2
  Math Function5/1 -> Sum7/2
  Math Function2/1 -> Sum7/1, Sum8/1
  Sum8/1 -> Saturation3/1
  Sum7/1 -> Saturation4/1
  Sqrt2/1 -> Saturation Dynamic2/1, Gain2/1
  Sqrt3/1 -> Saturation Dynamic3/1, Gain3/1
  "Q priority "/1 -> Switch4/2, Switch9/2
  [Qref] -> Switch9/1
  [PFV] -> Switch4/3
  [PpccPu] -> Math Function5/1
  Saturation3/1 -> Sqrt2/1
  Saturation4/1 -> Sqrt3/1
  Gain2/1 -> Saturation Dynamic2/3
  Gain3/1 -> Saturation Dynamic3/3
  [PFV] -> Saturation Dynamic2/2
  [Qref] -> Saturation Dynamic3/2
  Saturation Dynamic2/1 -> Switch4/1
  Saturation Dynamic3/1 -> Switch9/3
  Qref limits/1 -> Switch2/3

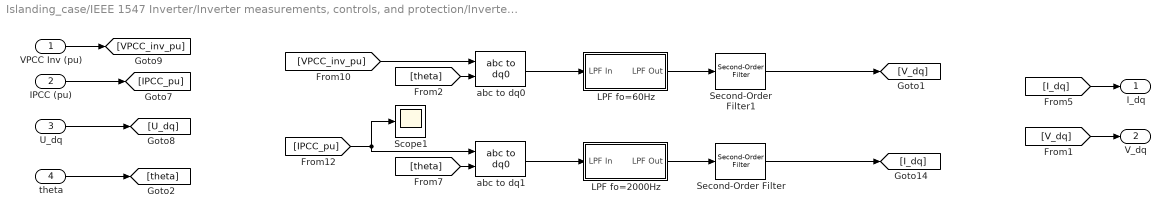
== system Islanding_case/IEEE 1547 Inverter/Inverter measurements, controls, and protection/Inverter control in positive sequence/abc to dq0  ==
  VPCC Inv (pu) : Inport
  IPCC (pu) : Inport  Port=2
  U_dq : Inport  Port=3
  theta : Inport  Port=4
  LPF fo=2000Hz : Subsystem  mask{f=2000}
      mask prompts: f "Cutoff Frequency (Hz)"
  LPF fo=60Hz : Subsystem  mask{f=NomFreq}
      mask prompts: f "Cutoff Frequency (Hz)"
  Scope1 : Scope
  Second-Order Filter : spsSecondOrderFilterLib/Second-Order Filter  FilterType=Bandstop (Notch)  Fo=120  Zeta=0.05  Ts=0  Initialize=on  Vac_Init="[0,  0,  NomFreq]"  Vdc_Init=0  PlotResponse=off  FreqRange=[0, 500, 1]
      settings: LibrarySourceBlock=|
      | sps_lib/Control/Filters/Second-Order
      | Filter
  Second-Order Filter1 : spsSecondOrderFilterLib/Second-Order Filter  FilterType=Bandstop (Notch)  Fo=120  Zeta=0.05  Ts=0  Initialize=on  Vac_Init="[0,  0,  NomFreq]"  Vdc_Init=0  PlotResponse=off  FreqRange=[0, 500, 1]
      settings: LibrarySourceBlock=|
      | sps_lib/Control/Filters/Second-Order
      | Filter
  abc to dq0 : spsabctodq0Lib/abc to dq0  Alignment=90 degrees behind phase A axis
  abc to dq1 : spsabctodq0Lib/abc to dq0  Alignment=90 degrees behind phase A axis
  I_dq : Outport  VectorParamsAs1DForOutWhenUnconnected=off
  V_dq : Outport  Port=2  VectorParamsAs1DForOutWhenUnconnected=off
  wires:
  Second-Order Filter1/1 -> [V_dq]
  Second-Order Filter/1 -> [I_dq]
  [theta] -> abc to dq1/2
  [theta] -> abc to dq0/2
  theta/1 -> [theta]
  abc to dq1/1 -> LPF fo=2000Hz/1(LPF In)
  LPF fo=60Hz/1(LPF Out) -> Second-Order Filter1/1
  abc to dq0/1 -> LPF fo=60Hz/1(LPF In)
  LPF fo=2000Hz/1(LPF Out) -> Second-Order Filter/1
  [IPCC_pu] -> Scope1/1, abc to dq1/1
  [VPCC_inv_pu] -> abc to dq0/1
  VPCC Inv (pu)/1 -> [VPCC_inv_pu]
  [I_dq] -> I_dq/1
  U_dq/1 -> [U_dq]
  IPCC (pu)/1 -> [IPCC_pu]
  [V_dq] -> V_dq/1
